simulink model "simuMotorFeedforward"  (R2014a)
settings: Solver=ode45  StartTime=0.0  StopTime=3  MaxStep=0.0001  RelTol=1e-3
values from neighbouring files (symbols this model uses):
  contr = param    [parametres.m]
undefined symbols (not defined in the file or in its folder): param
settings Model: Creator=Etienne  LastModifiedBy=Etienne

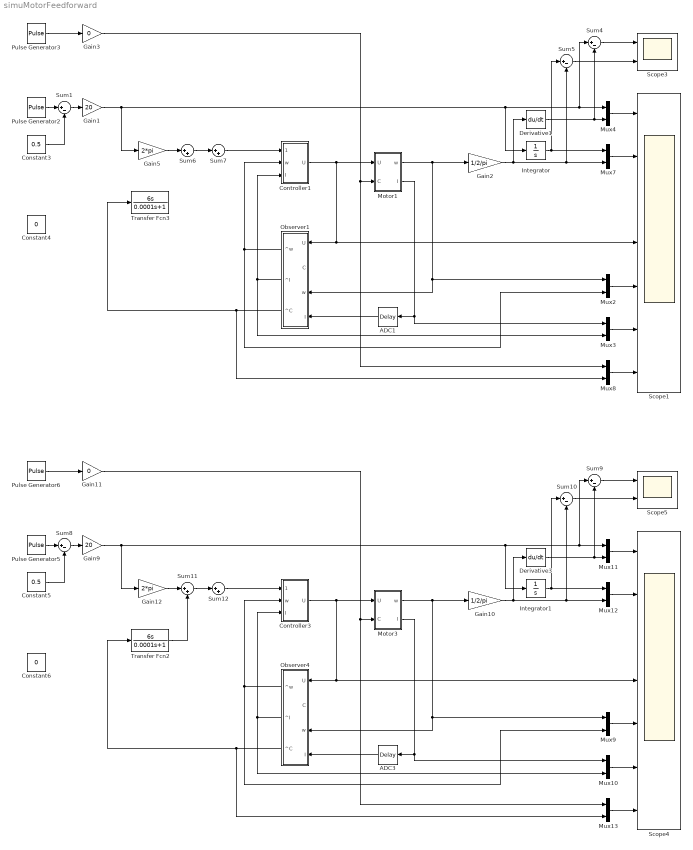
== system simuMotorFeedforward ==
  ADC1 : TransportDelay  DelayTime=78/2/param.fadc
  ADC3 : TransportDelay  DelayTime=78/2/144000
  Constant3 : Constant  Value=0.5
  Constant4 : Constant  Value=0
  Constant5 : Constant  Value=0.5
  Constant6 : Constant  Value=0
  Controller1 : Subsystem
  Controller3 : Subsystem
  Derivative1 : Derivative
  Derivative3 : Derivative
  Gain1 : Gain  Gain=20
  Gain10 : Gain  Gain=1/2/pi
  Gain11 : Gain  Gain=0
  Gain12 : Gain  Gain=2*pi
  Gain2 : Gain  Gain=1/2/pi
  Gain3 : Gain  Gain=0
  Gain5 : Gain  Gain=2*pi
  Gain9 : Gain  Gain=20
  Integrator : Integrator
  Integrator1 : Integrator
  Motor1 : Subsystem
  Motor3 : Subsystem
  Mux{2..4,7..13} (10 alike) : Mux  Inputs=2
  Observer1 : Subsystem
  Observer4 : Subsystem
  Pulse Generator2 : DiscretePulseGenerator  PulseType=Time based  Period=1  PulseWidth=50  PhaseDelay=0.25
  Pulse Generator3 : DiscretePulseGenerator  PulseType=Time based  Period=0.35  PulseWidth=50  PhaseDelay=0.3
  Pulse Generator5 : DiscretePulseGenerator  PulseType=Time based  Period=1  PulseWidth=50  PhaseDelay=0.25
  Pulse Generator6 : DiscretePulseGenerator  PulseType=Time based  Period=0.35  PulseWidth=50  PhaseDelay=0.3
  Scope1 : Scope  NumInputPorts=7
      settings: TimeRange=3  YMin=-20~-4~-1~-20~-20~-1~-1  YMax=20~4~1~20~20~1~1  SaveName=ScopeData2  MaxDataPoints=500000
  Scope3 : Scope  NumInputPorts=2
      settings: TimeRange=3  YMin=-25~-0.0025  YMax=25~0.0025  SaveName=ScopeData3  MaxDataPoints=500000
  Scope4 : Scope  NumInputPorts=7
      settings: TimeRange=3  YMin=-20~-4~-1~-20~-20~-1~-1  YMax=20~4~1~20~20~1~1  SaveName=ScopeData4  MaxDataPoints=500000
  Scope5 : Scope  NumInputPorts=2
      settings: TimeRange=3  YMin=-25~-0.0025  YMax=25~0.0025  SaveName=ScopeData5  MaxDataPoints=500000
  Sum{1,4..5,8..10} (6 alike) : Sum  Inputs=|+-
  Sum{6..7,11..12} (4 alike) : Sum  Inputs=|++
  Transfer Fcn2 : TransferFcn  Numerator=[6 0]  Denominator=[0.0001 1]
  Transfer Fcn3 : TransferFcn  Numerator=[6 0]  Denominator=[0.0001 1]
  wires:
  Pulse Generator3/1 -> Gain3/1
  Motor1/1(w) -> Gain2/1, Observer1/3(w), Mux2/1
  Motor1/2(I) -> Mux3/1, ADC1/1
  Pulse Generator2/1 -> Sum1/1
  Sum1/1 -> Gain1/1
  Constant3/1 -> Sum1/2
  Gain2/1 -> Sum5/2, Mux7/2, Derivative1/1
  Controller1/1(U) -> Scope1/4, Observer1/1(U), Motor1/1(U)
  ADC1/1 -> Observer1/4(I)
  Mux4/1 -> Scope1/1
  Observer1/1(^w) -> Controller1/2(w), Mux2/2
  Observer1/2(^I) -> Controller1/3(I), Mux3/2
  Observer1/3(^C) -> Transfer Fcn3/1, Mux8/2
  Gain1/1 -> Mux4/1, Sum4/1, Integrator/1, Gain5/1
  Gain3/1 -> Mux8/1, Motor1/2(C)
  Derivative1/1 -> Sum4/2, Mux4/2
  Mux7/1 -> Scope1/2
  Integrator/1 -> Mux7/1, Sum5/1
  Mux2/1 -> Scope1/5
  Mux3/1 -> Scope1/6
  Mux8/1 -> Scope1/7
  Sum4/1 -> Scope3/1
  Sum5/1 -> Scope3/2
  Sum7/1 -> Controller1/1(cons)
  Sum6/1 -> Sum7/1
  Gain5/1 -> Sum6/1
  Pulse Generator6/1 -> Gain11/1
  Motor3/1(w) -> Gain10/1, Observer4/3(w), Mux9/1
  Motor3/2(I) -> Mux10/1, ADC3/1
  Pulse Generator5/1 -> Sum8/1
  Sum8/1 -> Gain9/1
  Constant5/1 -> Sum8/2
  Gain10/1 -> Sum10/2, Mux12/2, Derivative3/1
  Controller3/1(U) -> Scope4/4, Observer4/1(U), Motor3/1(U)
  ADC3/1 -> Observer4/4(I)
  Mux11/1 -> Scope4/1
  Observer4/1(^w) -> Controller3/2(w), Mux9/2
  Observer4/2(^I) -> Controller3/3(I), Mux10/2
  Observer4/3(^C) -> Transfer Fcn2/1, Mux13/2
  Gain9/1 -> Mux11/1, Sum9/1, Integrator1/1, Gain12/1
  Gain11/1 -> Mux13/1, Motor3/2(C)
  Derivative3/1 -> Sum9/2, Mux11/2
  Mux12/1 -> Scope4/2
  Integrator1/1 -> Mux12/1, Sum10/1
  Mux9/1 -> Scope4/5
  Mux10/1 -> Scope4/6
  Mux13/1 -> Scope4/7
  Sum9/1 -> Scope5/1
  Sum10/1 -> Scope5/2
  Sum12/1 -> Controller3/1(cons)
  Sum11/1 -> Sum12/1
  Gain12/1 -> Sum11/1
  Transfer Fcn2/1 -> Sum11/2

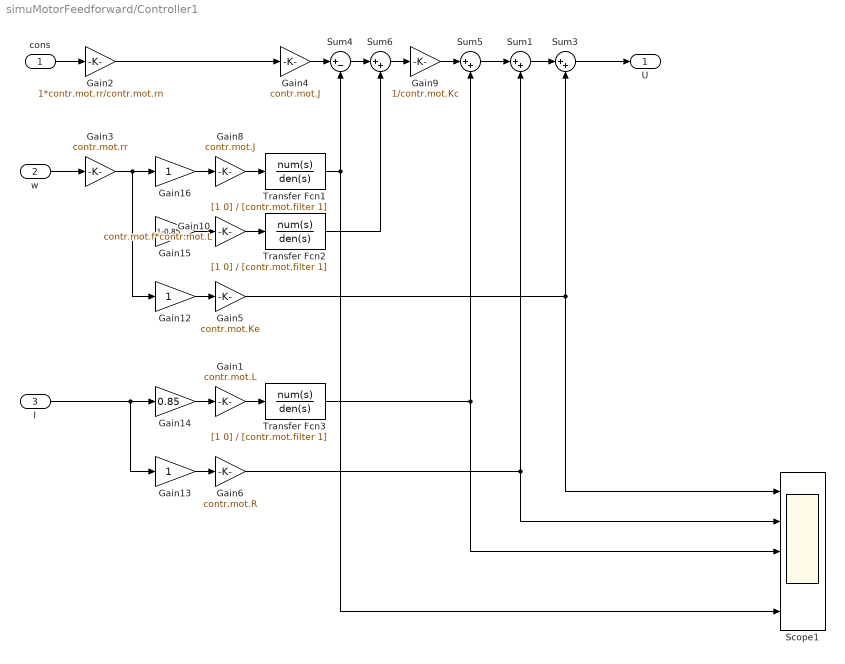
== system simuMotorFeedforward/Controller1 ==
  cons : Inport
  w : Inport  Port=2
  I : Inport  Port=3
  Gain1 : Gain  Gain=contr.mot.L
  Gain10 : Gain  Gain=contr.mot.f*contr.mot.L
  Gain12 : Gain
  Gain13 : Gain
  Gain14 : Gain  Gain=0.85
  Gain15 : Gain  Gain=1-0.85
  Gain16 : Gain
  Gain2 : Gain  Gain=1*contr.mot.rr/contr.mot.rn
  Gain3 : Gain  Gain=contr.mot.rr
  Gain4 : Gain  Gain=contr.mot.J
  Gain5 : Gain  Gain=contr.mot.Ke
  Gain6 : Gain  Gain=contr.mot.R
  Gain8 : Gain  Gain=contr.mot.J
  Gain9 : Gain  Gain=1/contr.mot.Kc
  Scope1 : Scope  NumInputPorts=5
      settings: TimeRange=10  YMin=-30~-5~-1~-1~-0.04  YMax=30~5~1~1~0.04  MaxDataPoints=500000
  Sum{1,3,5..6} (4 alike) : Sum  Inputs=|++
  Sum4 : Sum  Inputs=|+-
  Transfer Fcn1 : TransferFcn  Numerator=[1 0]  Denominator=[contr.mot.filter 1]
  Transfer Fcn2 : TransferFcn  Numerator=[1 0]  Denominator=[contr.mot.filter 1]
  Transfer Fcn3 : TransferFcn  Numerator=[1 0]  Denominator=[contr.mot.filter 1]
  U : Outport
  wires:
  Gain5/1 -> Scope1/1, Sum3/2
  Gain8/1 -> Transfer Fcn1/1
  Gain3/1 -> Gain16/1, Gain12/1
  Gain2/1 -> Gain4/1
  Sum1/1 -> Sum3/1
  Gain6/1 -> Scope1/2, Sum1/2
  Sum3/1 -> U/1
  Sum6/1 -> Gain9/1
  Transfer Fcn1/1 -> Scope1/5, Sum4/2
  Transfer Fcn3/1 -> Scope1/3, Sum5/2
  Sum5/1 -> Sum1/1
  Gain12/1 -> Gain5/1
  Gain9/1 -> Sum5/1
  Gain1/1 -> Transfer Fcn3/1
  Gain15/1 -> Gain10/1
  Gain16/1 -> Gain8/1
  Gain13/1 -> Gain6/1
  Gain14/1 -> Gain1/1
  Sum4/1 -> Sum6/1
  cons/1 -> Gain2/1
  w/1 -> Gain3/1
  I/1 -> Gain14/1, Gain13/1
  Gain4/1 -> Sum4/1
  Gain10/1 -> Transfer Fcn2/1
  Transfer Fcn2/1 -> Sum6/2

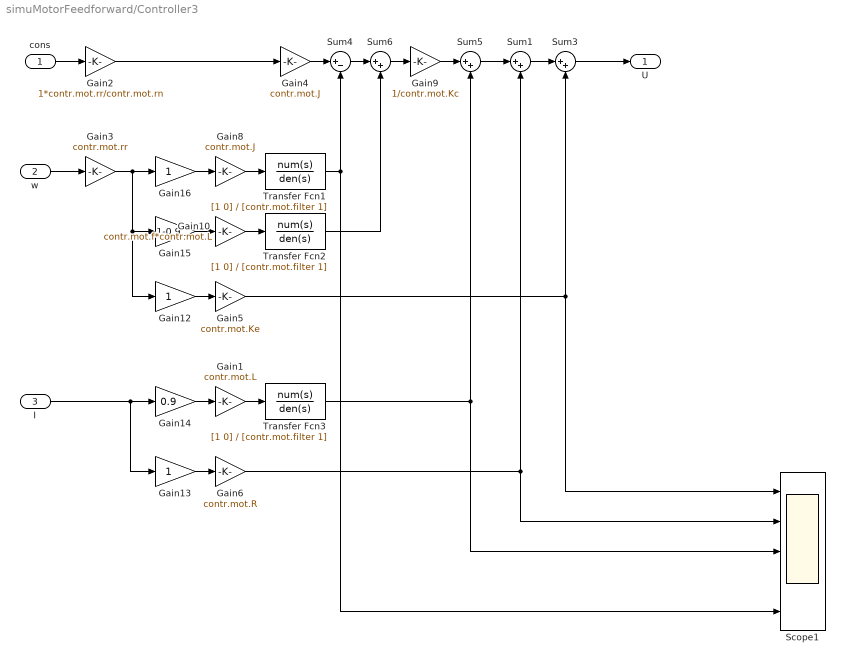
== system simuMotorFeedforward/Controller3 ==
  cons : Inport
  w : Inport  Port=2
  I : Inport  Port=3
  Gain1 : Gain  Gain=contr.mot.L
  Gain10 : Gain  Gain=contr.mot.f*contr.mot.L
  Gain12 : Gain
  Gain13 : Gain
  Gain14 : Gain  Gain=0.9
  Gain15 : Gain  Gain=1-0.9
  Gain16 : Gain
  Gain2 : Gain  Gain=1*contr.mot.rr/contr.mot.rn
  Gain3 : Gain  Gain=contr.mot.rr
  Gain4 : Gain  Gain=contr.mot.J
  Gain5 : Gain  Gain=contr.mot.Ke
  Gain6 : Gain  Gain=contr.mot.R
  Gain8 : Gain  Gain=contr.mot.J
  Gain9 : Gain  Gain=1/contr.mot.Kc
  Scope1 : Scope  NumInputPorts=5
      settings: TimeRange=10  YMin=-30~-5~-1~-1~-0.04  YMax=30~5~1~1~0.04  MaxDataPoints=500000
  Sum{1,3,5..6} (4 alike) : Sum  Inputs=|++
  Sum4 : Sum  Inputs=|+-
  Transfer Fcn1 : TransferFcn  Numerator=[1 0]  Denominator=[contr.mot.filter 1]
  Transfer Fcn2 : TransferFcn  Numerator=[1 0]  Denominator=[contr.mot.filter 1]
  Transfer Fcn3 : TransferFcn  Numerator=[1 0]  Denominator=[contr.mot.filter 1]
  U : Outport
  wires:
  Gain5/1 -> Scope1/1, Sum3/2
  Gain8/1 -> Transfer Fcn1/1
  Gain3/1 -> Gain16/1, Gain15/1, Gain12/1
  Gain2/1 -> Gain4/1
  Sum1/1 -> Sum3/1
  Gain6/1 -> Scope1/2, Sum1/2
  Sum3/1 -> U/1
  Sum6/1 -> Gain9/1
  Transfer Fcn1/1 -> Scope1/5, Sum4/2
  Transfer Fcn3/1 -> Scope1/3, Sum5/2
  Sum5/1 -> Sum1/1
  Gain12/1 -> Gain5/1
  Gain9/1 -> Sum5/1
  Gain1/1 -> Transfer Fcn3/1
  Gain15/1 -> Gain10/1
  Gain16/1 -> Gain8/1
  Gain13/1 -> Gain6/1
  Gain14/1 -> Gain1/1
  Sum4/1 -> Sum6/1
  cons/1 -> Gain2/1
  w/1 -> Gain3/1
  I/1 -> Gain13/1, Gain14/1
  Gain4/1 -> Sum4/1
  Gain10/1 -> Transfer Fcn2/1
  Transfer Fcn2/1 -> Sum6/2

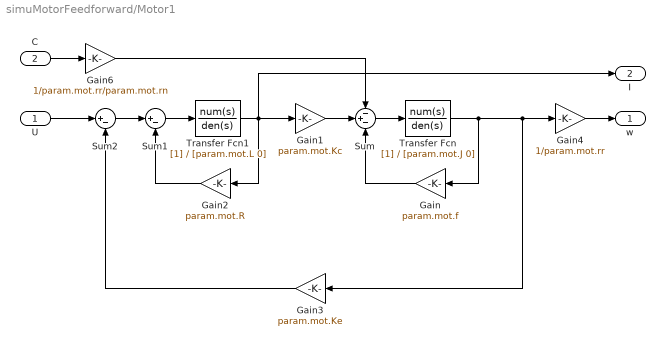
== system simuMotorFeedforward/Motor1 ==
  U : Inport
  C : Inport  Port=2
  Gain : Gain  Gain=param.mot.f
  Gain1 : Gain  Gain=param.mot.Kc
  Gain2 : Gain  Gain=param.mot.R
  Gain3 : Gain  Gain=param.mot.Ke
  Gain4 : Gain  Gain=1/param.mot.rr
  Gain6 : Gain  Gain=1/param.mot.rr/param.mot.rn
  Sum : Sum  Inputs=-+-
  Sum1 : Sum  Inputs=|+-
  Sum2 : Sum  Inputs=|+-
  Transfer Fcn : TransferFcn  Denominator=[param.mot.J 0]
  Transfer Fcn1 : TransferFcn  Denominator=[param.mot.L 0]
  w : Outport
  I : Outport  Port=2
  wires:
  Gain1/1 -> Sum/2
  Transfer Fcn/1 -> Gain3/1, Gain4/1, Gain/1
  Gain3/1 -> Sum2/2
  Gain/1 -> Sum/3
  Sum2/1 -> Sum1/1
  Gain2/1 -> Sum1/2
  Sum1/1 -> Transfer Fcn1/1
  U/1 -> Sum2/1
  C/1 -> Gain6/1
  Gain6/1 -> Sum/1
  Gain4/1 -> w/1
  Sum/1 -> Transfer Fcn/1
  Transfer Fcn1/1 -> Gain1/1, I/1, Gain2/1

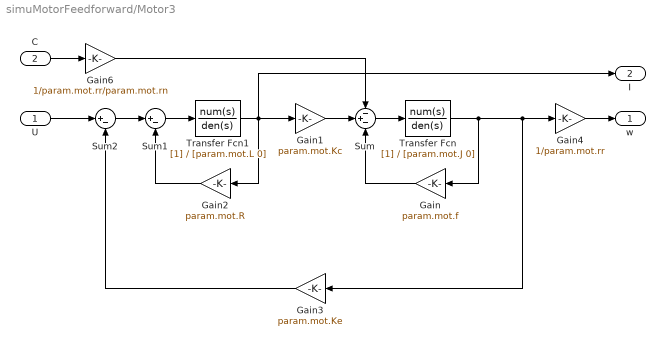
== system simuMotorFeedforward/Motor3 ==
  U : Inport
  C : Inport  Port=2
  Gain : Gain  Gain=param.mot.f
  Gain1 : Gain  Gain=param.mot.Kc
  Gain2 : Gain  Gain=param.mot.R
  Gain3 : Gain  Gain=param.mot.Ke
  Gain4 : Gain  Gain=1/param.mot.rr
  Gain6 : Gain  Gain=1/param.mot.rr/param.mot.rn
  Sum : Sum  Inputs=-+-
  Sum1 : Sum  Inputs=|+-
  Sum2 : Sum  Inputs=|+-
  Transfer Fcn : TransferFcn  Denominator=[param.mot.J 0]
  Transfer Fcn1 : TransferFcn  Denominator=[param.mot.L 0]
  w : Outport
  I : Outport  Port=2
  wires:
  Gain1/1 -> Sum/2
  Transfer Fcn/1 -> Gain3/1, Gain4/1, Gain/1
  Gain3/1 -> Sum2/2
  Gain/1 -> Sum/3
  Sum2/1 -> Sum1/1
  Gain2/1 -> Sum1/2
  Sum1/1 -> Transfer Fcn1/1
  U/1 -> Sum2/1
  C/1 -> Gain6/1
  Gain6/1 -> Sum/1
  Gain4/1 -> w/1
  Sum/1 -> Transfer Fcn/1
  Transfer Fcn1/1 -> Gain1/1, I/1, Gain2/1

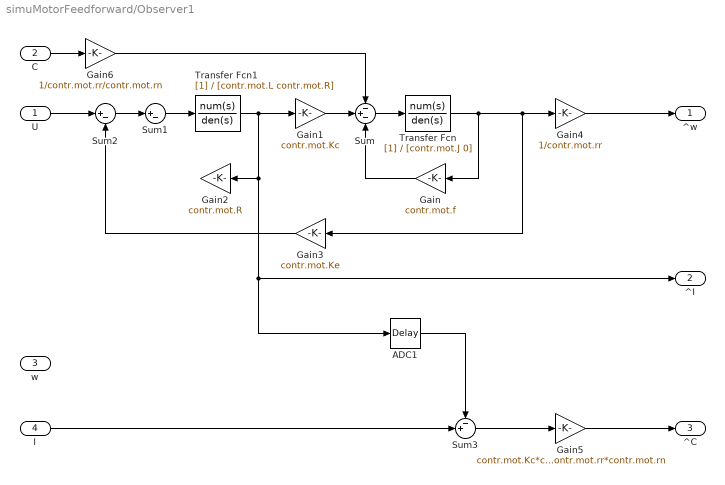
== system simuMotorFeedforward/Observer1 ==
  U : Inport
  C : Inport  Port=2
  w : Inport  Port=3
  I : Inport  Port=4
  ADC1 : TransportDelay  DelayTime=78/2/param.fadc
  Gain : Gain  Gain=contr.mot.f
  Gain1 : Gain  Gain=contr.mot.Kc
  Gain2 : Gain  Gain=contr.mot.R
  Gain3 : Gain  Gain=contr.mot.Ke
  Gain4 : Gain  Gain=1/contr.mot.rr
  Gain5 : Gain  Gain=contr.mot.Kc*contr.mot.rr*contr.mot.rn
  Gain6 : Gain  Gain=1/contr.mot.rr/contr.mot.rn
  Sum : Sum  Inputs=-+-
  Sum1 : Sum  Inputs=|+-
  Sum2 : Sum  Inputs=|+-
  Sum3 : Sum  Inputs=-+|
  Transfer Fcn : TransferFcn  Denominator=[contr.mot.J 0]
  Transfer Fcn1 : TransferFcn  Denominator=[contr.mot.L contr.mot.R]
  ^w : Outport
  ^I : Outport  Port=2
  ^C : Outport  Port=3
  wires:
  Gain1/1 -> Sum/2
  Transfer Fcn/1 -> Gain3/1, Gain4/1, Gain/1
  Gain3/1 -> Sum2/2
  Gain/1 -> Sum/3
  Sum2/1 -> Sum1/1
  Sum1/1 -> Transfer Fcn1/1
  U/1 -> Sum2/1
  C/1 -> Gain6/1
  Gain6/1 -> Sum/1
  Gain4/1 -> ^w/1
  Sum/1 -> Transfer Fcn/1
  Transfer Fcn1/1 -> ADC1/1, ^I/1, Gain2/1, Gain1/1
  Sum3/1 -> Gain5/1
  I/1 -> Sum3/2
  Gain5/1 -> ^C/1
  ADC1/1 -> Sum3/1

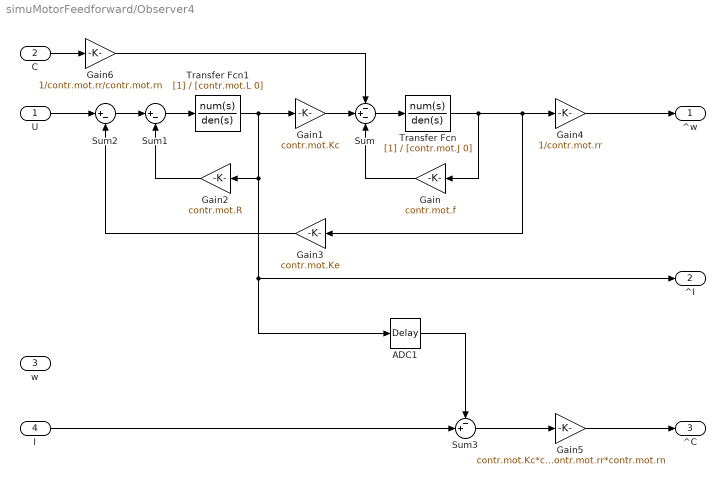
== system simuMotorFeedforward/Observer4 ==
  U : Inport
  C : Inport  Port=2
  w : Inport  Port=3
  I : Inport  Port=4
  ADC1 : TransportDelay  DelayTime=78/2/144000
  Gain : Gain  Gain=contr.mot.f
  Gain1 : Gain  Gain=contr.mot.Kc
  Gain2 : Gain  Gain=contr.mot.R
  Gain3 : Gain  Gain=contr.mot.Ke
  Gain4 : Gain  Gain=1/contr.mot.rr
  Gain5 : Gain  Gain=contr.mot.Kc*contr.mot.rr*contr.mot.rn
  Gain6 : Gain  Gain=1/contr.mot.rr/contr.mot.rn
  Sum : Sum  Inputs=-+-
  Sum1 : Sum  Inputs=|+-
  Sum2 : Sum  Inputs=|+-
  Sum3 : Sum  Inputs=-+|
  Transfer Fcn : TransferFcn  Denominator=[contr.mot.J 0]
  Transfer Fcn1 : TransferFcn  Denominator=[contr.mot.L 0]
  ^w : Outport
  ^I : Outport  Port=2
  ^C : Outport  Port=3
  wires:
  Gain1/1 -> Sum/2
  Transfer Fcn/1 -> Gain3/1, Gain4/1, Gain/1
  Gain3/1 -> Sum2/2
  Gain/1 -> Sum/3
  Sum2/1 -> Sum1/1
  Gain2/1 -> Sum1/2
  Sum1/1 -> Transfer Fcn1/1
  U/1 -> Sum2/1
  C/1 -> Gain6/1
  Gain6/1 -> Sum/1
  Gain4/1 -> ^w/1
  Sum/1 -> Transfer Fcn/1
  Transfer Fcn1/1 -> ADC1/1, ^I/1, Gain2/1, Gain1/1
  Sum3/1 -> Gain5/1
  I/1 -> Sum3/2
  Gain5/1 -> ^C/1
  ADC1/1 -> Sum3/1
